simulink model "gm_untitled1"  (R2021a)
settings: Solver=FixedStepAuto  StartTime=0.0  StopTime=10.0  RelTol=1e-3
libraries: dspsrcs4 x2, dspsnks4 x1, dspvision x1, dspadpt3 x1
settings Model: Creator=hanmengyuan  LastModifiedBy=hanmengyuan
settings OptimizationCC: BlockReduction=off  ConditionallyExecuteInputs=off  DefaultParameterBehavior=Inlined  OptimizeBlockIOStorage=off  EnhancedBackFolding=on  PassReuseOutputArgsThreshold=0  OptimizeDataStoreBuffers=off  BusAssignmentInplaceUpdate=off
settings DebuggingCC: AlgebraicLoopMsg=error  InheritedTsInSrcMsg=none  ParameterTunabilityLossMsg=error  SFUnexpectedBacktrackingDiag=warning  SFNoUnconditionalDefaultTransitionDiag=warning
settings HardwareCC: ProdBitPerPointer=32  ProdBitPerSizeT=32  ProdBitPerPtrDiffT=32  ProdLargestAtomicFloat=None  ProdIntDivRoundTo=Undefined  ProdEndianess=Unspecified  ProdWordSize=32  ProdHWDeviceType=ASIC/FPGA->ASIC/FPGA  TargetBitPerPointer=64  TargetBitPerSizeT=64  TargetBitPerPtrDiffT=64  TargetLongLongMode=on  TargetIntDivRoundTo=Zero  TargetEndianess=LittleEndian  TargetWordSize=64  TargetHWDeviceType=Custom Processor->MATLAB Host Computer  ProdEqTarget=off
settings SFSimCC: MATLABDynamicMemAlloc=off
settings RTWCC: Description=Generic Real-Time Target  GenerateReport=on  BuildConfiguration=Debug  LaunchReport=on
settings CodeAppCC: ForceParamTrailComments=on  OperatorAnnotations=on  MATLABSourceComments=on  EnableCustomComments=on
settings GRTTargetCC: CombineSignalStateStructs=on  SupportVariableSizeSignals=on  MultiInstanceErrorCode=Warning

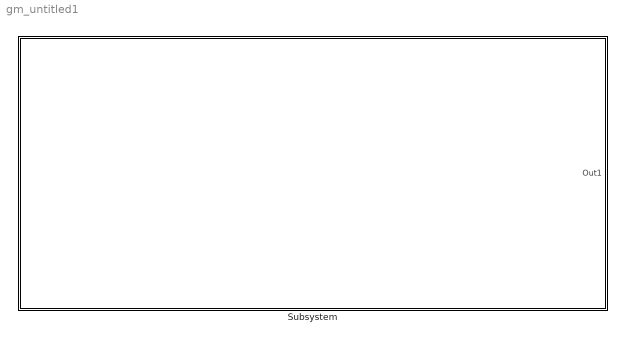
== system gm_untitled1 ==
  Subsystem : Subsystem

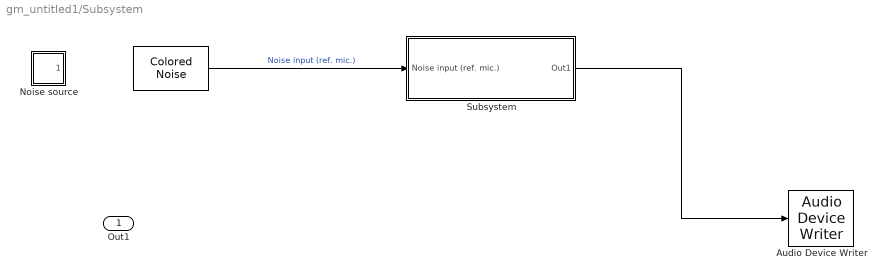
== system gm_untitled1/Subsystem ==
  " " : dspsrcs4/Colored Noise  Color=white  InverseFrequencyPower=1  BoundedOutput=off  NumChannels=1  OutputDataType=double  SamplesPerFrame=1  SampleTime=1/8820  RandomStream=mt19937ar with seed  Seed=67  SimulateUsing=Interpreted execution
      settings: SourceProductBaseCode=DS
  Audio Device Writer : dspsnks4/Audio Device Writer  Driver=DirectSound  Device=Default  InheritSampleRate=on  SampleRate=8000  BitDepth=16-bit integer  BufferSize=4096  NumBuffers=10  DefaultOutputChannelMapping=on  OutputChannelMapping=1:2  OutputNumUnderrunSamples=off  DriverIdx=1  DeviceWarnFlag=''
  Noise source : Subsystem
  Subsystem : Subsystem
  Out1 : Outport
  wires:
  " "/1 -> Subsystem/1(Noise input (ref. mic.))  "Noise input (ref. mic.)"
  Subsystem/1(Out1) -> Audio Device Writer/1

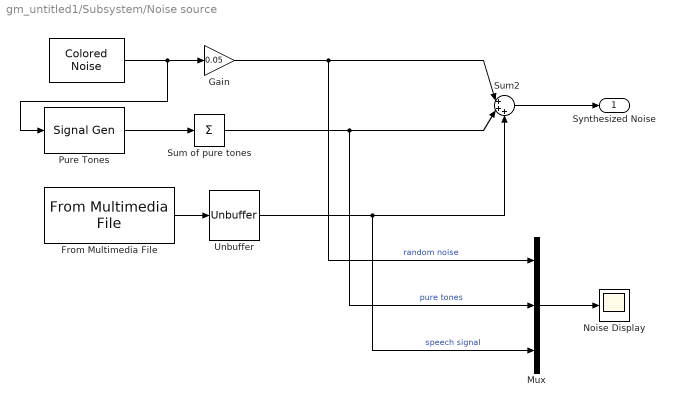
== system gm_untitled1/Subsystem/Noise source ==
  " " : dspsrcs4/Colored Noise  Color=white  InverseFrequencyPower=1  BoundedOutput=off  NumChannels=1  OutputDataType=double  SamplesPerFrame=1  SampleTime=1/8820  RandomStream=mt19937ar with seed  Seed=67  SimulateUsing=Interpreted execution
      settings: SourceProductBaseCode=DS
  From Multimedia File : dspvision/From Multimedia File  inputFilename=D:\各项文件\FPGA人声分离系统\主动降噪\speech3.wav  readRange=[1 Inf]  loop=on  numPlays=inf  outputStreams=Audio only  videoDataType=single  audioDataType=double  inheritSampleTime=on  userDefinedSampleTime=1/8820  noAudioOutput=off  isIntensityVideo=off  fourcc=RGB  colorVideoFormat=Separate color signals  outputEOF=off  dataOrg=Column-major  audioFrameSize=2048  computeAudioFrameSize=off  outSamplingMode=Sample based
  Gain : Gain  Gain=0.05
  Mux : Mux  Inputs=3
  Noise Display : Scope
  Pure Tones : SignalGenerator  TimeSource=Use external signal  Amplitude=0.03  Frequency=[30 2000]
  Sum of pure tones : Sum  Inputs=+
  Sum2 : Sum  Inputs=|+++
  Unbuffer : Unbuffer
  Synthesized Noise : Outport  VectorParamsAs1DForOutWhenUnconnected=off
  wires:
  From Multimedia File/1 -> Unbuffer/1
  Gain/1 -> Mux/1, Sum2/1  "random noise"
  Mux/1 -> Noise Display/1
  Sum of pure tones/1 -> Mux/2, Sum2/2  "pure tones"
  Sum2/1 -> Synthesized Noise/1
  " "/1 -> Pure Tones/1, Gain/1
  Pure Tones/1 -> Sum of pure tones/1
  Unbuffer/1 -> Mux/3, Sum2/3  "speech signal"

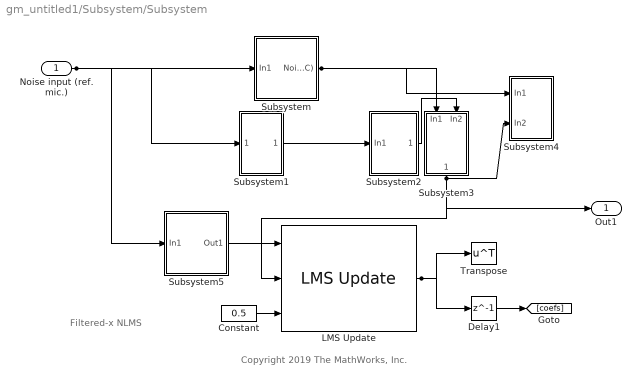
== system gm_untitled1/Subsystem/Subsystem ==
  note: Filtered-x NLMS
  note: Copyright 2019 The MathWorks, Inc.
  Noise input (ref. mic.) : Inport
  Constant : Constant  Value=0.5
  Delay1 : Delay  DelayLength=1
  LMS Update : dspadpt3/LMS Update  Method=Normalized LMS  Length=24  StepSizeSource=Input port  StepSize=0.1  LeakageFactor=1.0  InitialConditions=0  EnableAdaptInput=off  EnableResetInput=off  SimulateUsing=Interpreted execution
      settings: SourceProductBaseCode=DS
  Subsystem : Subsystem
  Subsystem1 : Subsystem
  Subsystem2 : Subsystem
  Subsystem3 : Subsystem
  Subsystem4 : Subsystem
  Subsystem5 : Subsystem
  Transpose : Math  Operator=transpose  SignedPower=on  SaturateOnIntegerOverflow=on
  Out1 : Outport
  wires:
  Subsystem5/1(Out1) -> LMS Update/1
  Subsystem2/1(Out1) -> Subsystem3/2(In2)
  Subsystem3/1(Error mic.) -> LMS Update/2, Out1/1, Subsystem4/2(In2)
  Subsystem1/1(Out1) -> Subsystem2/1(In1)
  Subsystem/1(Noise output (no ANC)) -> Subsystem3/1(In1), Subsystem4/1(In1)
  LMS Update/1 -> Delay1/1, Transpose/1
  Noise input (ref. mic.)/1 -> Subsystem1/1(In1), Subsystem5/1(In1), Subsystem/1(In1)
  Constant/1 -> LMS Update/3
  Delay1/1 -> [coefs]

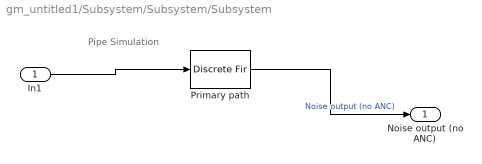
== system gm_untitled1/Subsystem/Subsystem/Subsystem ==
  note: Pipe Simulation
  In1 : Inport
  Primary path : DiscreteFir  Coefficients=conv([0.5 0.5 -.3 -.3 -.2 -.2],[.1 -.1 .2 -.2 .3 -.3 .15 -.15])
  Noise output (no ANC) : Outport
  wires:
  In1/1 -> Primary path/1
  Primary path/1 -> Noise output (no ANC)/1  "Noise output (no ANC)"

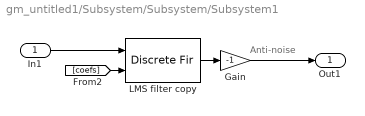
== system gm_untitled1/Subsystem/Subsystem/Subsystem1 ==
  note: Anti-noise
  In1 : Inport
  Gain : Gain  Gain=-1
  LMS filter copy : DiscreteFir  CoefSource=Input port
      settings: InputPortMap=u0,u1
  Out1 : Outport
  wires:
  LMS filter copy/1 -> Gain/1
  In1/1 -> LMS filter copy/1
  [coefs] -> LMS filter copy/2
  Gain/1 -> Out1/1

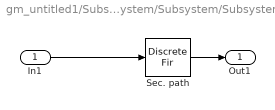
== system gm_untitled1/Subsystem/Subsystem/Subsystem2 ==
  In1 : Inport
  Sec. path : DiscreteFir  Coefficients=[0.5 0.5 -.3 -.3 -.2 -.2]
  Out1 : Outport
  wires:
  Sec. path/1 -> Out1/1
  In1/1 -> Sec. path/1

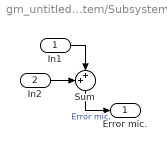
== system gm_untitled1/Subsystem/Subsystem/Subsystem3 ==
  In1 : Inport
  In2 : Inport  Port=2
  Sum : Sum  Inputs=++|
  Error mic. : Outport
  wires:
  In1/1 -> Sum/2
  Sum/1 -> Error mic./1  "Error mic."
  In2/1 -> Sum/1

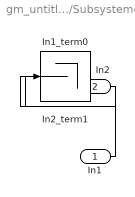
== system gm_untitled1/Subsystem/Subsystem/Subsystem4 ==
  In1 : Inport  OutDataTypeStr=double  PortDimensions=1  SampleTime=0.000113378684807256
  In2 : Inport  Port=2  OutDataTypeStr=double  PortDimensions=1  SampleTime=0.000113378684807256
  In1_term0 : Terminator
  In2_term1 : Terminator
  wires:
  In1/1 -> In1_term0/1
  In2/1 -> In2_term1/1

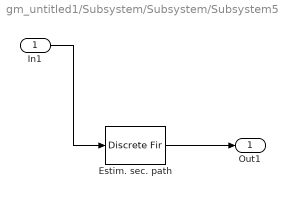
== system gm_untitled1/Subsystem/Subsystem/Subsystem5 ==
  In1 : Inport
  Estim. sec. path : DiscreteFir  Coefficients="[0.466  0.533  -0.257  -0.274  -0.231  -0.175]"
  Out1 : Outport
  wires:
  Estim. sec. path/1 -> Out1/1
  In1/1 -> Estim. sec. path/1
